simulink model "SimulationDroneSetup"  (R2025a)
settings: Solver=VariableStepAuto  StartTime=0.0  StopTime=10.0  RelTol=1e-3
settings Model: Creator=tobia  LastModifiedBy=dma

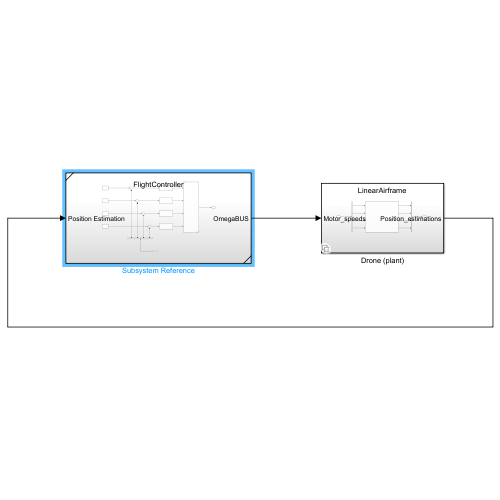
[thumbnail: Simulink's stored preview of the top-level diagram]
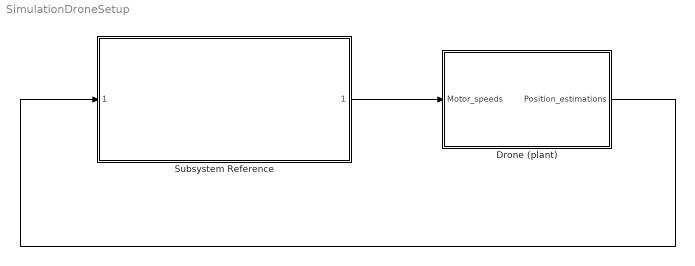
== system SimulationDroneSetup ==
  Drone (plant) : Subsystem  Variant=on
  Subsystem Reference : Subsystem  ReferencedSubsystem=FlightController
  wires:
  Subsystem Reference/1 -> Drone (plant)/1(Motor_speeds)
  Drone (plant)/1(Position_estimations) -> Subsystem Reference/1

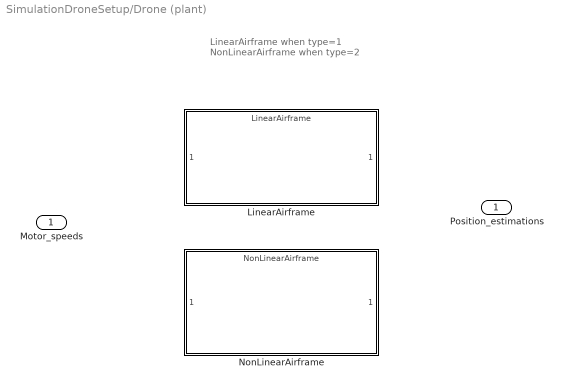
== system SimulationDroneSetup/Drone (plant) ==
  note: LinearAirframe when type=1
      | NonLinearAirframe when type=2
  Motor_speeds : Inport
  LinearAirframe : ModelReference  ModelNameDialog=LinearAirframe.slx  SimulationMode=Normal  VariantControl=type==1  ModelReferenceVersion=1.10
  NonLinearAirframe : ModelReference  ModelNameDialog=NonLinearAirframe.slx  SimulationMode=Normal  VariantControl=type==2  ModelReferenceVersion=1.4
  Position_estimations : Outport
